simulink model "battery_system_CV_PID"  (R2022a)
settings: Solver=VariableStepAuto  StartTime=0.0  StopTime=10.0  RelTol=1e-3
values from neighbouring files (symbols this model uses):
  AN = model.AN    [CV_Hold_main.m]    (also in CV_Hold_main_NoMultiple.m; CV_Hold_main_NoMultiple_Looped.m)
  C = C(1,:)    [CV_Hold_main.m]    (also in CV_Hold_main_NoMultiple.m = sys.C; CV_Hold_main_NoMultiple_Looped.m)
  CA = model.CA    [CV_Hold_main.m]    (also in CV_Hold_main_NoMultiple.m; CV_Hold_main_NoMultiple_Looped.m)
  CONS = model.CONS    [CV_Hold_main.m]    (also in CV_Hold_main_NoMultiple.m; CV_Hold_main_NoMultiple_Looped.m)
  Controller = pidtune(plant, 'PI', wc)    [CV_Hold_main_NoMultiple.m]    (also in CV_Hold_main_NoMultiple_Looped.m)
  CV = C*SV_IC    [CV_Hold_main.m]    (also in CV_Hold_main_NoMultiple.m; CV_Hold_main_NoMultiple_Looped.m)
  EL = model.EL    [CV_Hold_main.m]    (also in CV_Hold_main_NoMultiple.m; CV_Hold_main_NoMultiple_Looped.m)
  FLAG = model.FLAG    [CV_Hold_main.m]    (also in CV_Hold_main_NoMultiple.m; CV_Hold_main_NoMultiple_Looped.m)
  K_algb = diag(diag_vec)    [CV_Hold_main.m]    (also in CV_Hold_main_NoMultiple.m; CV_Hold_main_NoMultiple_Looped.m)
  M_cross = V*S_cross*U'    [CV_Hold_main.m]    (also in CV_Hold_main_NoMultiple.m; CV_Hold_main_NoMultiple_Looped.m)
  multiple = -SIM.A_c^-1    [CV_Hold_main_NoMultiple.m]
  N = model.N    [CV_Hold_main.m]    (also in CV_Hold_main_NoMultiple.m; CV_Hold_main_NoMultiple_Looped.m)
  P = model.P    [CV_Hold_main.m]    (also in CV_Hold_main_NoMultiple.m; CV_Hold_main_NoMultiple_Looped.m)
  PROPS = model.PROPS    [CV_Hold_main.m]    (also in CV_Hold_main_NoMultiple.m; CV_Hold_main_NoMultiple_Looped.m)
  SEP = model.SEP    [CV_Hold_main.m]    (also in CV_Hold_main_NoMultiple.m; CV_Hold_main_NoMultiple_Looped.m)
  SIM = rmfield(SIM,'fsolve_options')    [CV_Hold_main.m]    (also in CV_Hold_main_NoMultiple.m = rmfield(SIM,'Controller_MO_File'); CV_Hold_main_NoMultiple_Looped.m = rmfield(SIM,'Controller_MO_File'))
  SV_IC = model.SV_soln(end,:)'    [CV_Hold_main.m]    (also in CV_Hold_main_NoMultiple.m; CV_Hold_main_NoMultiple_Looped.m)
  U_NV_NT = U_null*V_null'    [CV_Hold_main.m]    (also in CV_Hold_main_NoMultiple.m; CV_Hold_main_NoMultiple_Looped.m)
settings Model: Creator=tyevans  LastModifiedBy=tyevans

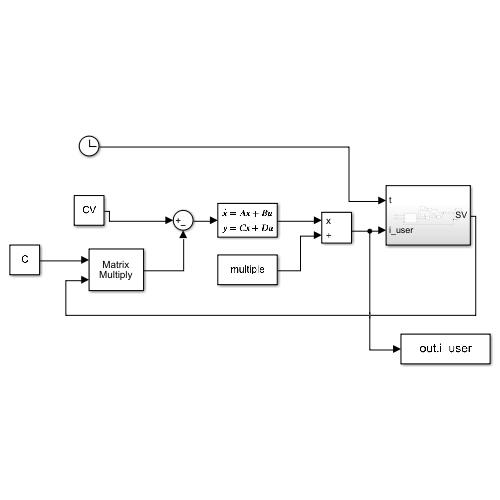
[thumbnail: Simulink's stored preview of the top-level diagram]
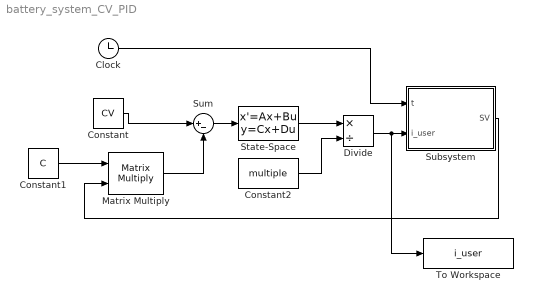
== system battery_system_CV_PID ==
  Clock : Clock
  Constant : Constant  Value=CV  VectorParams1D=off
  Constant1 : Constant  Value=C  VectorParams1D=off
  Constant2 : Constant  Value=multiple  VectorParams1D=off
  Divide : Product  Inputs=*/
  Matrix Multiply : Product  Multiplication=Matrix(*)
  State-Space : StateSpace  A=Controller.A  B=Controller.B  C=Controller.C  D=Controller.D  InitialCondition=0
  Subsystem : Subsystem
  Sum : Sum  Inputs=|+-
  To Workspace : ToWorkspace  VariableName=i_user  SampleTime=-1
      settings: Save2DSignal=2-D array (concatenate along first dimension)
  wires:
  Clock/1 -> Subsystem/1(t)
  Constant/1 -> Sum/1
  Constant1/1 -> Matrix Multiply/1
  Matrix Multiply/1 -> Sum/2
  Subsystem/1(SV) -> Matrix Multiply/2
  Constant2/1 -> Divide/2
  State-Space/1 -> Divide/1
  Divide/1 -> To Workspace/1, Subsystem/2(i_user)
  Sum/1 -> State-Space/1

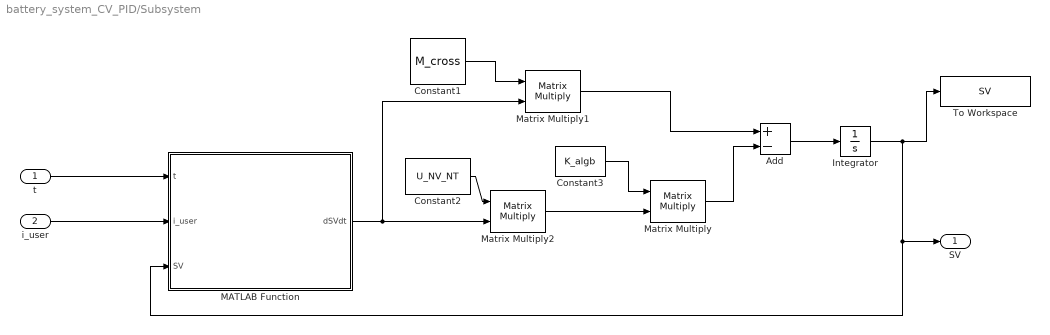
== system battery_system_CV_PID/Subsystem ==
  t : Inport
  i_user : Inport  Port=2
  Add : Sum  Inputs=+-
  Constant1 : Constant  Value=M_cross  VectorParams1D=off
  Constant2 : Constant  Value=U_NV_NT  VectorParams1D=off
  Constant3 : Constant  Value=K_algb  VectorParams1D=off
  Integrator : Integrator  InitialCondition=SV_IC
  MATLAB Function : MATLAB Function  TreatAsAtomicUnit=on
  Matrix Multiply : Product  Multiplication=Matrix(*)
  Matrix Multiply1 : Product  Multiplication=Matrix(*)
  Matrix Multiply2 : Product  Multiplication=Matrix(*)
  To Workspace : ToWorkspace  VariableName=SV  SampleTime=-1
  SV : Outport
  wires:
  Add/1 -> Integrator/1
  t/1 -> MATLAB Function/1(t)
  Matrix Multiply/1 -> Add/2
  Constant3/1 -> Matrix Multiply/1
  Constant1/1 -> Matrix Multiply1/1
  Constant2/1 -> Matrix Multiply2/1
  Matrix Multiply1/1 -> Add/1
  MATLAB Function/1(dSVdt) -> Matrix Multiply2/2, Matrix Multiply1/2
  Matrix Multiply2/1 -> Matrix Multiply/2
  Integrator/1 -> SV/1, MATLAB Function/3(SV), To Workspace/1
  i_user/1 -> MATLAB Function/2(i_user)

== matlab function battery_system_CV_PID/Subsystem/MATLAB Function ==
  data: t input; i_user input; dSVdt output; SV input; AN parameter; CA parameter; SEP parameter; EL parameter; SIM parameter; CONS parameter; P parameter; N parameter; FLAG parameter; PROPS parameter
function dSVdt = CallGovnEqns(t,i_user,SV, AN, CA, SEP, EL, SIM, CONS, P, N, FLAG, PROPS)
% Initialize Output
dSVdt = zeros(N.N_SV_tot,1);

% Call GovnEqns
coder.extrinsic('ConvertStrCallGov')
[dSVdt] = ConvertStrCallGov(t,SV,AN,CA,SEP,EL,SIM,CONS,P,N,FLAG,PROPS,i_user);

end
